simulink model "tgt_model"  (R2015a)
settings: configuration reference "config_cosim" (kept outside this file)
undefined symbols (not defined in the file): dsm_trj_tgt, one_new_tgt, pos, vel
libraries: simulink x1, Sys_CMD x1
settings Model: CovModelRefEnable=off  Creator=The MathWorks, Inc.  LastModifiedBy=ericli
settings ConfigSetRef: SourceLocation=Base Workspace

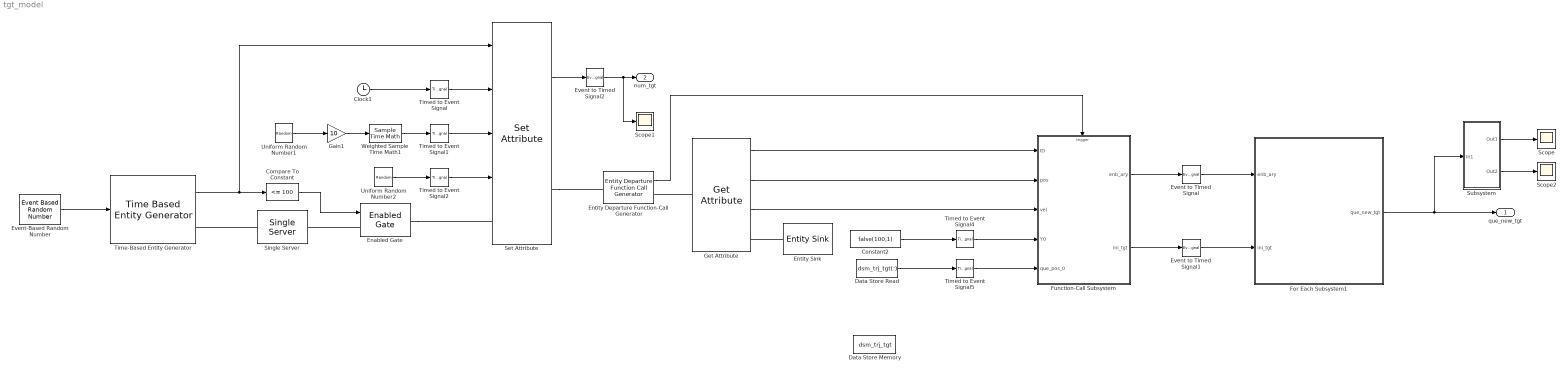
== system tgt_model ==
  Clock1 : Clock
  Compare To Constant : simulink/Logic and Bit Operations/Compare To Constant  relop=<=  const=100  OutDataTypeStr=boolean
  Constant2 : Constant  Value=false(100,1)
  Data Store Memory : DataStoreMemory  DataStoreName=dsm_trj_tgt  ReadBeforeWriteMsg=warning  WriteAfterWriteMsg=warning  WriteAfterReadMsg=warning  InitialValue=one_tgt  OutDataTypeStr=Bus: bus_trj_tgt  Dimensions=100
  Data Store Read : DataStoreRead  DataStoreName=dsm_trj_tgt  DataStoreElements=dsm_trj_tgt(:)
  Enabled Gate : EnabledGate
  Entity Departure Function-Call Generator : EntityDepartureFunctionCallGenerator
  Entity Sink : EntitySink
  Event to Timed Signal : EventToTimedSignal
  Event to Timed Signal1 : EventToTimedSignal
  Event to Timed Signal2 : EventToTimedSignal
  Event-Based Random Number : EventBasedRandomNumber  Distribution=Uniform  maxUnif=50  Seed=982145
  For Each Subsystem1 : Subsystem  TreatAsAtomicUnit=on
  Function-Call Subsystem : Subsystem  TreatAsAtomicUnit=on
  Gain1 : Gain  Gain=10
  Get Attribute : GetAttribute  AttributeName=ID|pos|vel  AttributeMissing=Error|Error|Error  AttributeDefaultValue=1|1|1  AttributeTreatAsVector=1|1|1  AttributeSendTiming=After entity departure|After entity departure|After entity departure  EvaluatedDefaultAttributeValue={ [];[];[]}
      settings: OutputPortMap=o1,o2,o3
  Scope : Scope
      settings: YMin=0  YMax=400
  Scope1 : Scope
  Scope2 : Scope
      settings: YMin=0  YMax=400  SaveName=ScopeData2
  Set Attribute : SetAttribute  AttributeName=ID|time|pos|vel  AttributeFrom=Signal port|Signal port|Signal port|Signal port  AttributeValue=1|1|1|1  AttributeTreatAsVector=1|1|1|1  StatNumberDeparted=on  EvaluatedAttributeValue={ [];[];[];[]}
      settings: InputPortMap=u0,u1,u2,u3
  Single Server : SingleServer  ServiceTime=0
  Subsystem : Subsystem
  Time-Based Entity Generator : TimeBasedEntityGenerator  GenerateEntitiesUpon=Intergeneration time from port t  GenerateEntityAtSimulationStart=off  StatNumberDeparted=on
  Timed to Event Signal{,1..2,4..5} (5 alike) : TimedToEventSignal
  Uniform Random Number1 : UniformRandomNumber  Minimum=[0 0 0]  Maximum=[1 1 1]  Seed=[854697 25478 362145]
  Uniform Random Number2 : UniformRandomNumber  Minimum=[-500 -500 -500]  Maximum=[500 500 500]  Seed=[12358 95471 26584]
  Weighted Sample Time Math1 : SampleTimeMath  weightValue=100
  que_new_tgt : Outport  OutDataTypeStr=Bus: bus_new_tgt  PortDimensions=100  BusOutputAsStruct=on
  num_tgt : Outport  Port=2
  wires:
  Subsystem/1(Out1) -> Scope/1
  Time-Based Entity Generator/1 -> Compare To Constant/1, Set Attribute/1
  Clock1/1 -> Timed to Event Signal/1
  Uniform Random Number1/1 -> Gain1/1
  Gain1/1 -> Weighted Sample Time Math1/1
  Weighted Sample Time Math1/1 -> Timed to Event Signal1/1
  Entity Departure Function-Call Generator/1 -> Function-Call Subsystem/Trigger
  Get Attribute/1 -> Function-Call Subsystem/1(ID)
  Get Attribute/2 -> Function-Call Subsystem/2(pos)
  Get Attribute/3 -> Function-Call Subsystem/3(vel)
  Constant2/1 -> Timed to Event Signal4/1
  Function-Call Subsystem/1(enb_ary) -> Event to Timed Signal/1
  Function-Call Subsystem/2(ini_tgt) -> Event to Timed Signal1/1
  Timed to Event Signal/1 -> Set Attribute/2
  Timed to Event Signal1/1 -> Set Attribute/3
  Uniform Random Number2/1 -> Timed to Event Signal2/1
  Timed to Event Signal4/1 -> Function-Call Subsystem/4(Y0)
  Timed to Event Signal5/1 -> Function-Call Subsystem/5(que_pos_0)
  Event to Timed Signal/1 -> For Each Subsystem1/1(enb_ary)
  Event to Timed Signal1/1 -> For Each Subsystem1/2(ini_tgt)
  Set Attribute/1 -> Event to Timed Signal2/1
  Event-Based Random Number/1 -> Time-Based Entity Generator/1
  Data Store Read/1 -> Timed to Event Signal5/1
  Compare To Constant/1 -> Enabled Gate/1
  Timed to Event Signal2/1 -> Set Attribute/4
  For Each Subsystem1/1(que_new_tgt) -> que_new_tgt/1, Subsystem/1(In1)
  Event to Timed Signal2/1 -> num_tgt/1, Scope1/1
  Subsystem/2(Out2) -> Scope2/1
  connections:
  Enabled Gate/RConn1 -- Set Attribute/LConn1
  Set Attribute/RConn1 -- Entity Departure Function-Call Generator/LConn1
  Get Attribute/LConn1 -- Entity Departure Function-Call Generator/RConn1
  Entity Sink/LConn1 -- Get Attribute/RConn1
  Enabled Gate/LConn1 -- Single Server/RConn1
  Single Server/LConn1 -- Time-Based Entity Generator/RConn1

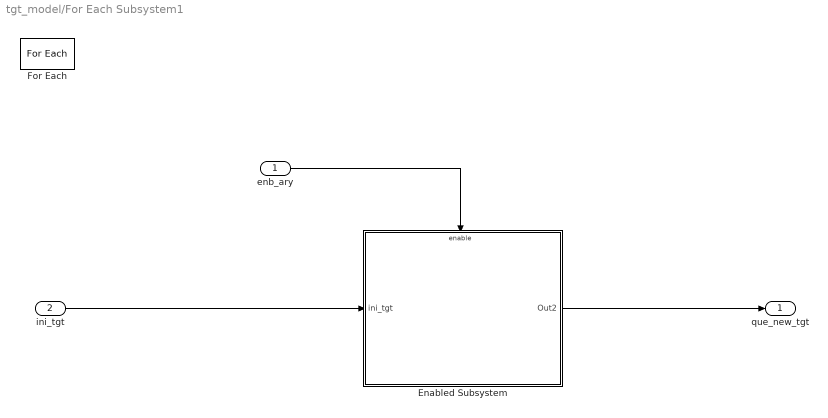
== system tgt_model/For Each Subsystem1 ==
  enb_ary : Inport  Partition=on  PartitionDimension=1  PartitionWidth=1
  ini_tgt : Inport  Port=2  OutDataTypeStr=Bus: bus_trj_tgt  PortDimensions=100  Partition=on  PartitionDimension=1  PartitionWidth=1
  Enabled Subsystem : Subsystem  TreatAsAtomicUnit=on
  For Each : ForEach  DisableCoverage=on  IndexMode=One-based
  que_new_tgt : Outport  OutDataTypeStr=Bus: bus_new_tgt  ConcatenationDimension=1
  wires:
  Enabled Subsystem/1(Out2) -> que_new_tgt/1
  enb_ary/1 -> Enabled Subsystem/Enable
  ini_tgt/1 -> Enabled Subsystem/1(ini_tgt)

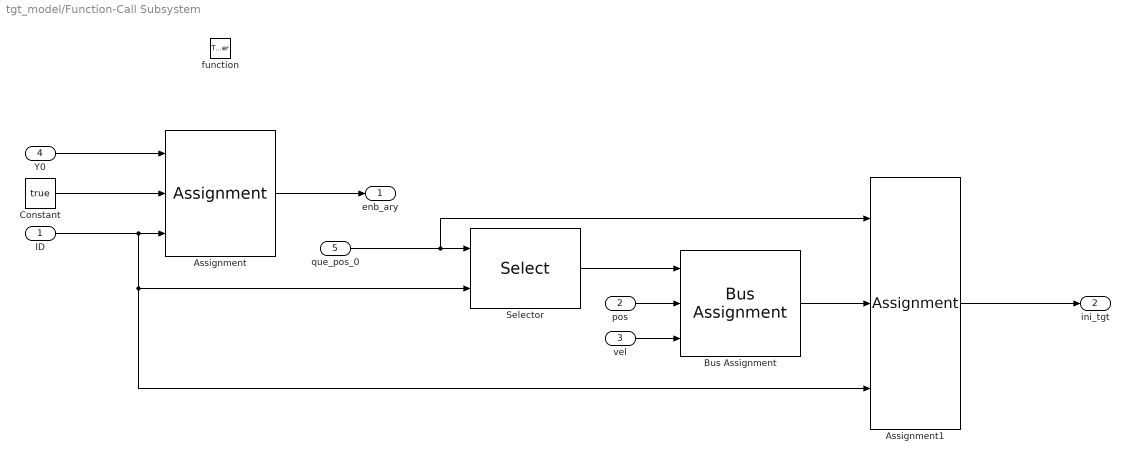
== system tgt_model/Function-Call Subsystem ==
  ID : Inport
  pos : Inport  Port=2  PortDimensions=3
  vel : Inport  Port=3  PortDimensions=3
  Y0 : Inport  Port=4  OutDataTypeStr=boolean  PortDimensions=[100,1]
  que_pos_0 : Inport  Port=5  OutDataTypeStr=Bus: bus_trj_tgt
  function : TriggerPort  TriggerType=function-call
  Assignment : Assignment  DiagnosticForDimensions=Warning  IndexOptions=Index vector (port)
  Assignment1 : Assignment  DiagnosticForDimensions=Warning  IndexOptions=Index vector (port)
  Bus Assignment : BusAssignment  AssignedSignals=pos,vel
  Constant : Constant  Value=true
  Selector : Selector  InputPortWidth=100  IndexOptions=Index vector (port)  Indices=[1 3]
  enb_ary : Outport
  ini_tgt : Outport  Port=2  OutDataTypeStr=Bus: bus_trj_tgt
  wires:
  Y0/1 -> Assignment/1
  Constant/1 -> Assignment/2
  ID/1 -> Assignment1/3, Selector/2, Assignment/3
  Assignment/1 -> enb_ary/1
  que_pos_0/1 -> Assignment1/1, Selector/1
  pos/1 -> Bus Assignment/2
  vel/1 -> Bus Assignment/3
  Selector/1 -> Bus Assignment/1
  Bus Assignment/1 -> Assignment1/2
  Assignment1/1 -> ini_tgt/1

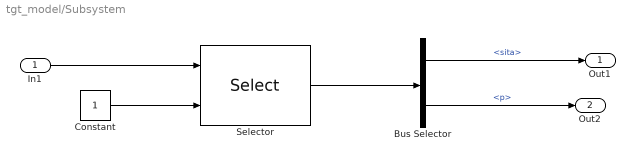
== system tgt_model/Subsystem ==
  In1 : Inport
  Bus Selector : BusSelector  OutputSignals=sita,p
  Constant : Constant
  Selector : Selector  InputPortWidth=100  IndexOptions=Index vector (port)  Indices=[1 3]
  Out1 : Outport
  Out2 : Outport  Port=2
  wires:
  Bus Selector/1 -> Out1/1  "<sita>"
  Constant/1 -> Selector/2
  Selector/1 -> Bus Selector/1
  In1/1 -> Selector/1
  Bus Selector/2 -> Out2/1  "<p>"

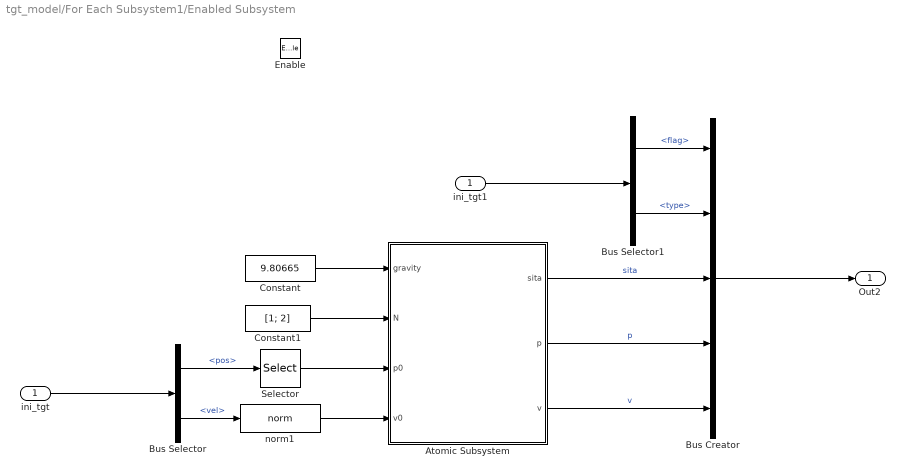
== system tgt_model/For Each Subsystem1/Enabled Subsystem ==
  ini_tgt : Inport  OutDataTypeStr=Bus: bus_trj_tgt
  Enable : EnablePort
  Atomic Subsystem : Subsystem  TreatAsAtomicUnit=on
  Bus Creator : BusCreator  Inputs=5  OutDataTypeStr=Bus: bus_new_tgt  NonVirtualBus=on
  Bus Selector : BusSelector  OutputSignals=pos,vel
  Bus Selector1 : BusSelector  OutputSignals=flag,type
  Constant : Constant  Value=9.80665
  Constant1 : Constant  Value=[1; 2]
  Selector : Selector  InputPortWidth=3  Indices=[1 2]
  ini_tgt1 : InportShadow  OutDataTypeStr=Bus: bus_trj_tgt
  norm1 : Sys_CMD/norm
  Out2 : Outport  OutDataTypeStr=Bus: bus_new_tgt  InitialOutput=one_new_tgt
  wires:
  Atomic Subsystem/3(v) -> Bus Creator/5  "v"
  Atomic Subsystem/2(p) -> Bus Creator/4  "p"
  Atomic Subsystem/1(sita) -> Bus Creator/3  "sita"
  Bus Selector1/2 -> Bus Creator/2  "<type>"
  Bus Selector1/1 -> Bus Creator/1  "<flag>"
  ini_tgt1/1 -> Bus Selector1/1
  norm1/1 -> Atomic Subsystem/4(v0)
  Selector/1 -> Atomic Subsystem/3(p0)
  Bus Selector/2 -> norm1/1  "<vel>"
  Bus Selector/1 -> Selector/1  "<pos>"
  Constant1/1 -> Atomic Subsystem/2(N)
  Constant/1 -> Atomic Subsystem/1(gravity)
  ini_tgt/1 -> Bus Selector/1
  Bus Creator/1 -> Out2/1

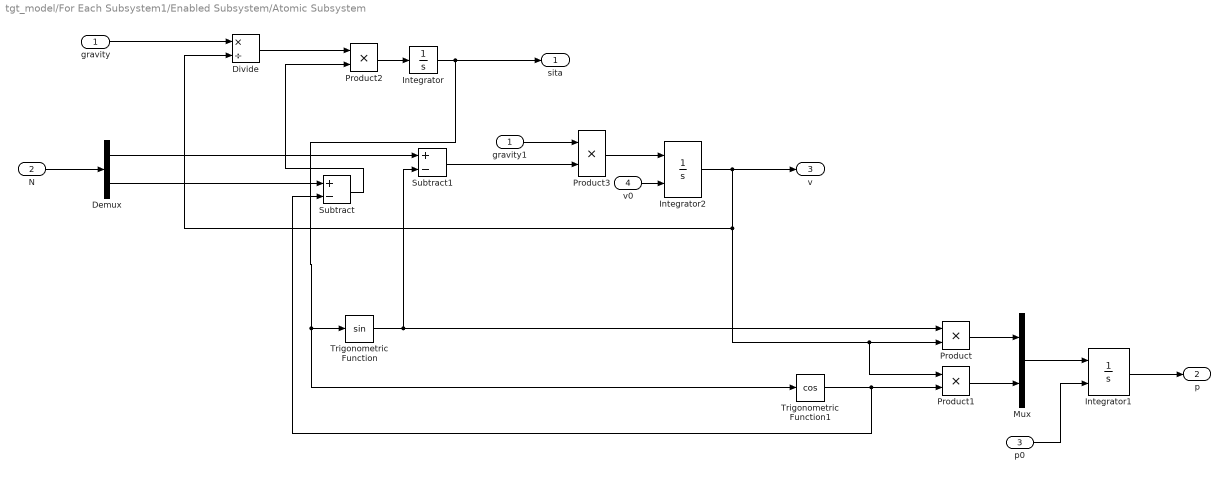
== system tgt_model/For Each Subsystem1/Enabled Subsystem/Atomic Subsystem ==
  gravity : Inport
  N : Inport  Port=2
  p0 : Inport  Port=3
  v0 : Inport  Port=4
  Demux : Demux  Outputs=2
  Divide : Product  Inputs=*/
  Integrator : Integrator
  Integrator1 : Integrator  InitialConditionSource=external
  Integrator2 : Integrator  InitialConditionSource=external  InitialCondition=0.1
  Mux : Mux  Inputs=2
  Product{,1..3} (4 alike) : Product
  Subtract : Sum  Inputs=+-
  Subtract1 : Sum  Inputs=+-
  Trigonometric Function : Trigonometry
  Trigonometric Function1 : Trigonometry  Operator=cos
  gravity1 : InportShadow
  sita : Outport
  p : Outport  Port=2
  v : Outport  Port=3
  wires:
  v0/1 -> Integrator2/2
  p0/1 -> Integrator1/2
  gravity1/1 -> Product3/1
  Subtract1/1 -> Product3/2
  Product3/1 -> Integrator2/1
  Demux/1 -> Subtract1/1
  Product2/1 -> Integrator/1
  Subtract/1 -> Product2/2
  Demux/2 -> Subtract/1
  Divide/1 -> Product2/1
  N/1 -> Demux/1
  gravity/1 -> Divide/1
  Mux/1 -> Integrator1/1
  Product1/1 -> Mux/2
  Product/1 -> Mux/1
  Trigonometric Function1/1 -> Product1/2, Subtract/2
  Integrator2/1 -> v/1, Product/2, Product1/1, Divide/2
  Trigonometric Function/1 -> Product/1, Subtract1/2
  Integrator1/1 -> p/1
  Integrator/1 -> sita/1, Trigonometric Function/1, Trigonometric Function1/1
